simulink model "DT_Risk_Aware_MPC"  (R2025b)
settings: Solver=FixedStepAuto  StartTime=0.0  StopTime=Tsim  FixedStep=Ts  RelTol=1e-3
settings Model: Creator=HP  LastModifiedBy=HP

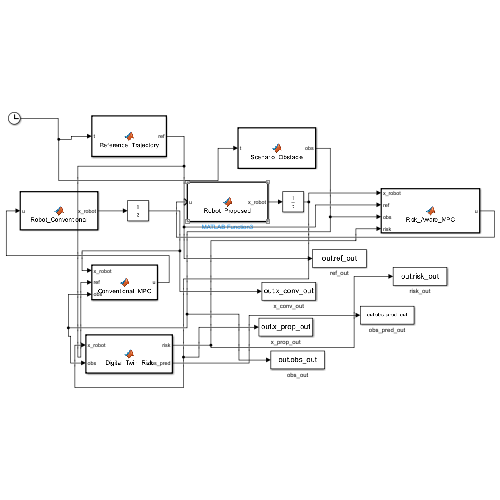
[thumbnail: Simulink's stored preview of the top-level diagram]
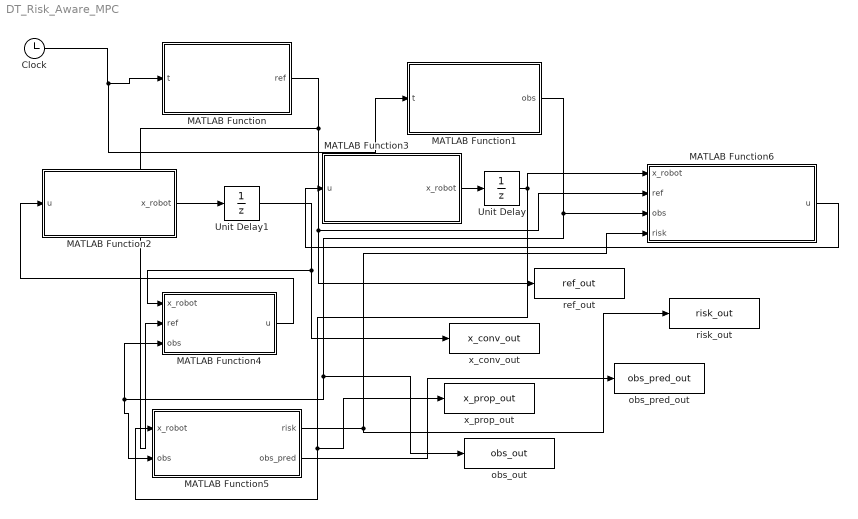
== system DT_Risk_Aware_MPC ==
  Clock : Clock
  MATLAB Function : MATLAB Function  TreatAsAtomicUnit=on
  MATLAB Function1 : MATLAB Function  TreatAsAtomicUnit=on
  MATLAB Function2 : MATLAB Function  TreatAsAtomicUnit=on
  MATLAB Function3 : MATLAB Function  TreatAsAtomicUnit=on
  MATLAB Function4 : MATLAB Function  TreatAsAtomicUnit=on
  MATLAB Function5 : MATLAB Function  TreatAsAtomicUnit=on
  MATLAB Function6 : MATLAB Function  TreatAsAtomicUnit=on
  Unit Delay : UnitDelay  InitialCondition=[0;2;0]  SampleTime=0.1  HasFrameUpgradeWarning=on
  Unit Delay1 : UnitDelay  InitialCondition=[0;2;0]  SampleTime=0.1  HasFrameUpgradeWarning=on
  obs_out : ToWorkspace  VariableName=obs_out  SaveFormat=Structure With Time  SampleTime=-1
  obs_pred_out : ToWorkspace  VariableName=obs_pred_out  SaveFormat=Structure With Time  SampleTime=-1
  ref_out : ToWorkspace  VariableName=ref_out  SaveFormat=Structure With Time  SampleTime=-1
  risk_out : ToWorkspace  VariableName=risk_out  SaveFormat=Structure With Time  SampleTime=-1
  x_conv_out : ToWorkspace  VariableName=x_conv_out  SaveFormat=Structure With Time  SampleTime=-1
  x_prop_out : ToWorkspace  VariableName=x_prop_out  SaveFormat=Structure With Time  SampleTime=-1
  wires:
  Clock/1 -> MATLAB Function1/1(t), MATLAB Function/1(t)
  MATLAB Function/1(ref) -> MATLAB Function6/2(ref), ref_out/1, MATLAB Function4/2(ref)
  MATLAB Function1/1(obs) -> MATLAB Function6/3(obs), MATLAB Function4/3(obs), MATLAB Function5/2(obs), obs_out/1
  MATLAB Function2/1(x_robot) -> Unit Delay1/1
  MATLAB Function4/1(u) -> MATLAB Function2/1(u)
  MATLAB Function3/1(x_robot) -> Unit Delay/1
  MATLAB Function5/1(risk) -> risk_out/1, MATLAB Function6/4(risk)
  MATLAB Function6/1(u) -> MATLAB Function3/1(u)
  MATLAB Function5/2(obs_pred) -> obs_pred_out/1
  Unit Delay1/1 -> x_conv_out/1, MATLAB Function4/1(x_robot)
  Unit Delay/1 -> MATLAB Function6/1(x_robot), x_prop_out/1, MATLAB Function5/1(x_robot)

== matlab function DT_Risk_Aware_MPC/MATLAB Function1 ==
  data: t input; obs output double size=[4 1]
function obs = Scenario_Obstacle(t)
% Environmental Obstacle Generator
obs = zeros(4,1);

% Scenario Selector:
% 1 = Obstacle-free
% 2 = Static obstacles
% 3 = Dynamic multi-obstacle clutter
scenario = 3;

if scenario == 1
    xo = 100.0; yo = 100.0; vox = 0.0; voy = 0.0;
elseif scenario == 2
    xo = 3.5; yo = 1.2; vox = 0.0; voy = 0.0;
else
    % Dynamic crossing obstacle trajectory matching Section VI-C
    xo = 2.8 + 0.04 * t;
    yo = 0.8 + 0.035 * t;
    vox = 0.04;
    voy = 0.035;
end

obs(1) = xo;
obs(2) = yo;
obs(3) = vox;
obs(4) = voy;
end

== matlab function DT_Risk_Aware_MPC/MATLAB Function ==
  data: t input; ref output double size=[3 1]
function ref = Reference_Trajectory(t)

% Explicit output size
ref = zeros(3,1);

x_ref = 0.12*t;
y_ref = 2*sin(0.12*t) + 2;
theta_ref = atan2(0.24*cos(0.12*t), 0.12);

ref(1) = x_ref;
ref(2) = y_ref;
ref(3) = theta_ref;

end

== matlab function DT_Risk_Aware_MPC/MATLAB Function2 ==
  data: u input double size=[2 1]; x_robot output double size=[3 1]
function x_robot = Robot_Conventional(u)

% Explicit output size
x_robot = zeros(3,1);

Ts = 0.1;

persistent x y theta

if isempty(x)
    x = 0;
    y = 2;
    theta = 0;
end

v = u(1);
w = u(2);

x = x + v*cos(theta)*Ts;
y = y + v*sin(theta)*Ts;
theta = theta + w*Ts;

x_robot(1) = x;
x_robot(2) = y;
x_robot(3) = theta;

end

== matlab function DT_Risk_Aware_MPC/MATLAB Function3 ==
  data: u input double size=[2 1]; x_robot output double size=[3 1]
function x_robot = Robot_Proposed(u)
% Kinematic Model for Proposed Robot (Nonholonomic Unicycle)
x_robot = zeros(3,1);
Ts = 0.1;

persistent x y theta
if isempty(x)
    x = 0;
    y = 2.0;
    theta = 0;
end

v = u(1);
w = u(2);

% Discrete Forward Euler Integration (Eqs. 6-8)
x = x + v * cos(theta) * Ts;
y = y + v * sin(theta) * Ts;
theta = theta + w * Ts;

x_robot(1) = x;
x_robot(2) = y;
x_robot(3) = theta;
end

== matlab function DT_Risk_Aware_MPC/MATLAB Function4 ==
  data: x_robot input double size=[3 1]; u output double size=[2 1]; ref input double size=[3 1]; obs input double size=[4 1]
function u = Conventional_MPC(x_robot, ref, obs)

% Explicit output size for Simulink
u = zeros(2,1);

vmax = 1.0;
wmax = 1.0;

x = x_robot(1);
y = x_robot(2);
theta = x_robot(3);

xr = ref(1);
yr = ref(2);

xo = obs(1);
yo = obs(2);

ex = xr - x;
ey = yr - y;

theta_d = atan2(ey, ex);
e_theta = atan2(sin(theta_d-theta), cos(theta_d-theta));
e_pos = sqrt(ex^2 + ey^2);

v = 0.8*e_pos;
w = 1.8*e_theta;

d = sqrt((x-xo)^2 + (y-yo)^2);

if d < 1.5
    avoid_angle = atan2(y-yo, x-xo);
    desired = 0.75*theta_d + 0.25*avoid_angle;
    e_avoid = atan2(sin(desired-theta), cos(desired-theta));
    w = 1.8*e_avoid;
end

v = min(max(v,0),vmax);
w = min(max(w,-wmax),wmax);

u(1) = v;
u(2) = w;

end

== matlab function DT_Risk_Aware_MPC/MATLAB Function5 ==
  data: x_robot input double size=[3 1]; risk output double size=[1 1]; obs input double size=[4 1]; obs_pred output double size=[2 20]
function [risk, obs_pred] = Digital_Twin_Risk(x_robot, obs)
% Digital Twin Future Obstacle Prediction & Collision-Risk Function
% Synchronized with Manuscript Section IV-C & IV-D (Eqs. 15-19)

risk = 0;
obs_pred = zeros(2,20);

Ts = 0.1;
Np = 20;
sigma = 0.35; % Risk sensitivity parameter (Table I)

x = x_robot(1);
y = x_robot(2);

xo  = obs(1);
yo  = obs(2);
vox = obs(3);
voy = obs(4);

risk_total = 0;

for i = 1:Np
    % Constant-Velocity Forward Trajectory Prediction (Eqs. 15-16)
    xo_pred = xo + vox * i * Ts;
    yo_pred = yo + voy * i * Ts;
    
    obs_pred(1,i) = xo_pred;
    obs_pred(2,i) = yo_pred;
    
    % Predicted Robot-Obstacle Distance (Eq. 17)
    d_i = sqrt((x - xo_pred)^2 + (y - yo_pred)^2);
    
    % Gaussian Risk Evaluation (Eq. 18)
    Gamma_i = exp(-(d_i^2) / (sigma^2));
    
    % Cumulative Horizon Risk (Eq. 19)
    risk_total = risk_total + Gamma_i;
end

risk = risk_total;
end

== matlab function DT_Risk_Aware_MPC/MATLAB Function6 ==
  data: x_robot input double size=[3 1]; u output double size=[2 1]; ref input double size=[3 1]; obs input double size=[4 1]; risk input double size=[1 1]
function u = Risk_Aware_MPC(x_robot, ref, obs, risk)
% Risk-Aware MPC Controller Function Block
% Synchronized with Manuscript Table I & System Model

u = zeros(2,1);

% Physical Constraints from Table I
vmax = 1.0;          % m/s
vmin = 0.0;          % m/s
wmax = 1.5;          % rad/s
wmin = -1.5;         % rad/s
d_safe = 0.250;      % m

% Current States
x = x_robot(1);
y = x_robot(2);
theta = x_robot(3);

xr = ref(1);
yr = ref(2);

xo = obs(1);
yo = obs(2);

% Tracking Errors
ex = xr - x;
ey = yr - y;
theta_d = atan2(ey, ex);
e_theta = atan2(sin(theta_d - theta), cos(theta_d - theta));
e_pos = sqrt(ex^2 + ey^2);

% Baseline Proportional Commands
v = 0.8 * e_pos;
w = 1.8 * e_theta;

% Repulsive Potential Guidance under Dynamic Risk
d = sqrt((x - xo)^2 + (y - yo)^2);
if d < (d_safe + 0.35)
    avoid_angle = atan2(y - yo, x - xo);
    desired_theta = 0.70 * theta_d + 0.30 * avoid_angle;
    e_avoid = atan2(sin(desired_theta - theta), cos(desired_theta - theta));
    w = 2.2 * e_avoid;
end

% Risk-aware speed modulation
v = v / (1 + 0.15 * risk);

% Actuator Saturations (Table I)
if v > vmax
    v = vmax;
elseif v < vmin
    v = vmin;
end

if w > wmax
    w = wmax;
elseif w < wmin
    w = wmin;
end

u(1) = v;
u(2) = w;
end
